simulink model "noisy_id_simulink"  (R2025a)
settings: Solver=VariableStepAuto  StartTime=0.0  StopTime=10.0  RelTol=1e-3
values from neighbouring files (symbols this model uses):
  w = W(i)    [noisy_id.m]
undefined symbols (not defined in the file or in its folder): noiseT
libraries: simulink x1
settings Model: Creator=USER  LastModifiedBy=USER

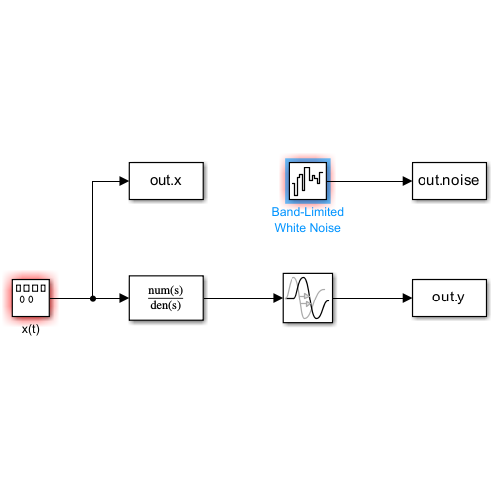
[thumbnail: Simulink's stored preview of the top-level diagram]
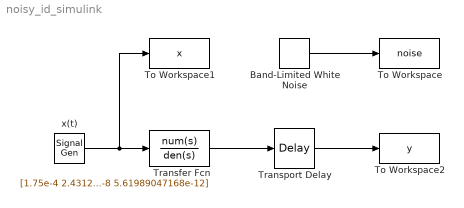
== system noisy_id_simulink ==
  Band-Limited White Noise : simulink/Sources/Band-Limited White Noise  Cov=noise_percentage  Ts=noiseT  seed=[23341]
  To Workspace : ToWorkspace  VariableName=noise  SaveFormat=Timeseries  SampleTime=-1
  To Workspace1 : ToWorkspace  VariableName=x  SaveFormat=Timeseries  SampleTime=-1
  To Workspace2 : ToWorkspace  VariableName=y  SaveFormat=Timeseries  SampleTime=-1
  Transfer Fcn : TransferFcn  Numerator=[1.75e-4 2.431275e-7 9.284625e-12]  Denominator=[1 3.87704e-2 2.551212584e-4 8.784303992e-8 5.61989047168e-12]
  Transport Delay : TransportDelay  DelayTime=9.3  BufferSize=2048
  x(t) : SignalGenerator  Frequency=w  Units=rad/sec
  wires:
  Transfer Fcn/1 -> Transport Delay/1
  x(t)/1 -> To Workspace1/1, Transfer Fcn/1
  Transport Delay/1 -> To Workspace2/1
  Band-Limited White Noise/1 -> To Workspace/1
